simulink model "Receive_Ethernet_UDP_2023a"  (R2024a)
settings: Solver=ode4  StartTime=0.0  StopTime=inf  FixedStep=0.01  RelTol=1e-3
undefined symbols (not defined in the file): f, gray
libraries: instrumentlib x2, etargetslib x1
settings Model: Creator=hyeon-yongjeong  LastModifiedBy=LG gram 17 - HW dev

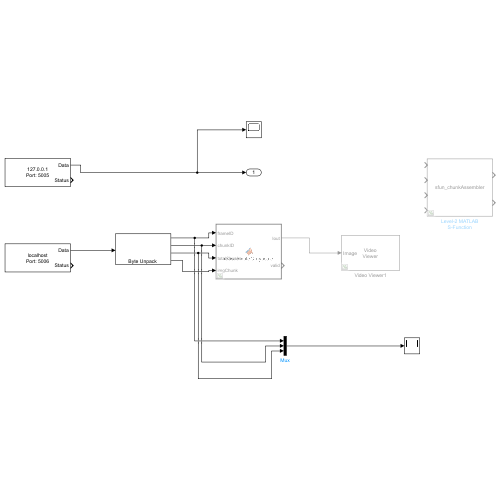
[thumbnail: Simulink's stored preview of the top-level diagram]
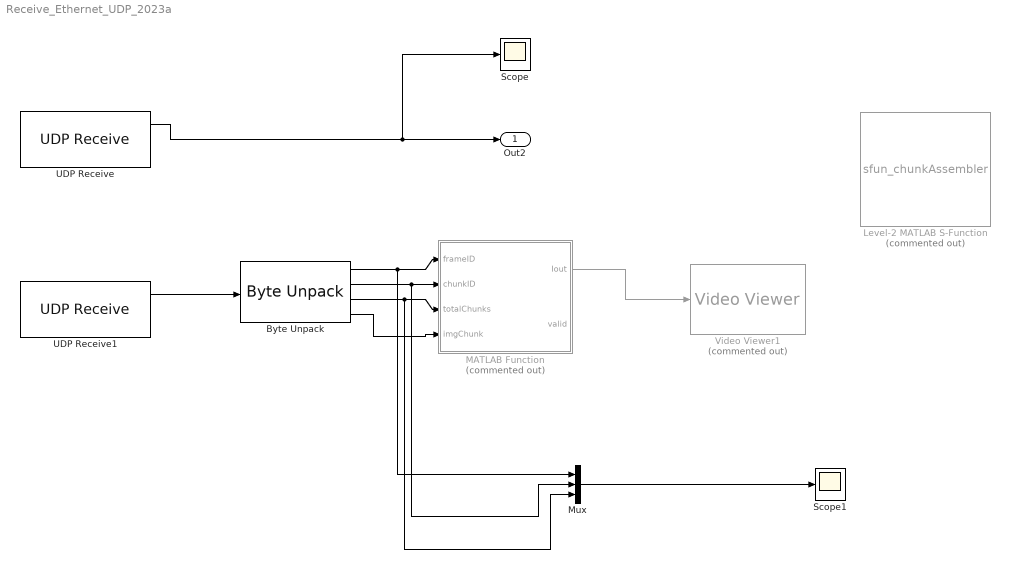
== system Receive_Ethernet_UDP_2023a ==
  Byte Unpack : etargetslib/Byte Unpack  dimensions="{[1 1],   [1 1],   [1 1],   [8192 1]}"  datatypes={'single', 'single', 'single', 'uint8'}  byteAlign=1
      settings: LibrarySourceBlock=embeddedtargetslib/Host Communication/Byte Unpack
  Level-2 MATLAB S-Function : M-S-Function  Commented=on  FunctionName=sfun_chunkAssembler
  MATLAB Function : MATLAB Function  Commented=on  TreatAsAtomicUnit=on
  Mux : Mux  Inputs=3
  Scope : Scope
  Scope1 : Scope
  UDP Receive : instrumentlib/UDP Receive  LocalAddress=127.0.0.1  LocalPort=5005  EnablePortSharing=off  Host=0.0.0.0  Port=5005  GetLatestData=off  DataSize=[6 1]  DataType=single  ASCIIFormatting=%f,  Terminator=LF  CustomTerminator=10  ByteOrder=little-endian  EnableBlockingMode=off  Timeout=10  SampleTime=0.01  SimulateUsing=Interpreted execution
  UDP Receive1 : instrumentlib/UDP Receive  LocalAddress=localhost  LocalPort=5006  EnablePortSharing=off  Host=0.0.0.0  Port=5006  GetLatestData=off  DataSize=[8192+4*3 1]  DataType=uint8  ASCIIFormatting=%f,  Terminator=LF  CustomTerminator=10  ByteOrder=big-endian  EnableBlockingMode=off  Timeout=10  SampleTime=-1  SimulateUsing=Interpreted execution
  Video Viewer1 : VideoViewer  Commented=on  colormapValue=gray(256)  FigPos=[107 926 636 450]
  Out2 : Outport
  wires:
  UDP Receive/1 -> Scope/1, Out2/1
  Byte Unpack/4 -> MATLAB Function/4(imgChunk)
  UDP Receive1/1 -> Byte Unpack/1
  MATLAB Function/1(Iout) -> Video Viewer1/1
  Byte Unpack/1 -> Mux/1, MATLAB Function/1(frameID)
  Byte Unpack/2 -> Mux/2, MATLAB Function/2(chunkID)
  Byte Unpack/3 -> Mux/3, MATLAB Function/3(totalChunks)
  Mux/1 -> Scope1/1

== matlab function Receive_Ethernet_UDP_2023a/MATLAB Function ==
  data: frameID input; Iout output; chunkID input; totalChunks input; imgChunk input; valid output
function [Iout, valid] = reassembleGrayscale(frameID, chunkID, totalChunks, imgChunk)
%#codegen
% Fixed image parameters
CHAN_H          = 480;
CHAN_W          = 640;
BYTES_PER_FRAME = CHAN_H * CHAN_W;           % 307200
CHUNK_SIZE      = 8192;                     % must match python
MAX_CHUNKS      = ceil(BYTES_PER_FRAME/CHUNK_SIZE);  % 38

% Persistent state
persistent prevID buf recCount recMask
if isempty(prevID)
    prevID   = uint32(0xFFFFFFFF);
    buf       = zeros(BYTES_PER_FRAME,1,'uint8');
    recCount  = uint16(0);
    recMask   = false(MAX_CHUNKS,1);
end

% New frame? reset everything
if frameID ~= prevID
    prevID    = frameID;
    buf(:)    = 0;
    recCount  = uint16(0);
    recMask(:)= false;
end

% Convert to doubles for arithmetic
dCID = double(chunkID);
dTC  = double(totalChunks);

% GUARD: skip any chunkID or totalChunks that’s nonsense
if dCID < 0 || dTC < 1 || dTC > MAX_CHUNKS || dCID >= dTC
    Iout  = zeros(CHAN_H, CHAN_W, 'uint8');
    valid = false;
    return;
end

% Compute how many bytes this chunk really contains
if dCID < dTC - 1
    nbytes = CHUNK_SIZE;
else
    nbytes = BYTES_PER_FRAME - CHUNK_SIZE*(dTC - 1);
end

% Copy only the valid portion into the buffer
offset = dCID * CHUNK_SIZE;  % zero‐based
buf(offset+1 : offset + nbytes) = imgChunk(1:nbytes);

% Mark this chunk as received
idx = dCID + 1;  % 1‐based index
if ~recMask(idx)
    recMask(idx) = true;
    recCount     = recCount + uint16(1);
end

% If we’ve got all chunks, assemble; otherwise blank
if recCount == totalChunks
    % reshape into [480×640] (col-major → row-major)
    Iout  = reshape(buf, CHAN_W, CHAN_H)';  
    valid = true;
else
    Iout  = zeros(CHAN_H, CHAN_W, 'uint8');
    valid = false;
end
end
